simulink model "LogisticDelayed2"  (Simulink 6.6)
settings: Solver=ode45  StartTime=0.0  StopTime=60  RelTol=1e-3
settings Model: Creator=mxkana  LastModifiedBy=mxkana

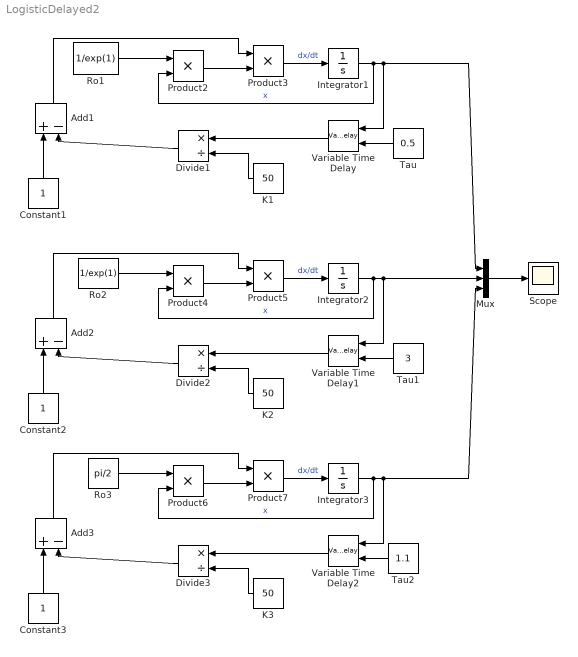
== system LogisticDelayed2 ==
  Add1 : Sum  Orientation=up  Inputs=+-  OutScaling=2^-10
  Add2 : Sum  Orientation=up  Inputs=+-  OutScaling=2^-10
  Add3 : Sum  Orientation=up  Inputs=+-  OutScaling=2^-10
  Constant1 : Constant  Orientation=up
  Constant2 : Constant  Orientation=up
  Constant3 : Constant  Orientation=up
  Divide1 : Product  Orientation=left  Inputs=*/  OutScaling=2^-10
  Divide2 : Product  Orientation=left  Inputs=*/  OutScaling=2^-10
  Divide3 : Product  Orientation=left  Inputs=*/  OutScaling=2^-10
  Integrator1 : Integrator  InitialCondition=1
  Integrator2 : Integrator  InitialCondition=1
  Integrator3 : Integrator  InitialCondition=1
  K1 : Constant  Orientation=left  Value=50
  K2 : Constant  Orientation=left  Value=50
  K3 : Constant  Orientation=left  Value=50
  Mux : Mux  Inputs=3
  Product{2..7} (6 alike) : Product  RndMeth=Zero
  Ro1 : Constant  Value=1/exp(1)
  Ro2 : Constant  Value=1/exp(1)
  Ro3 : Constant  Value=pi/2
  Scope : Scope
      settings: YMin=0  YMax=100
  Tau : Constant  Orientation=left  Value=0.5
  Tau1 : Constant  Orientation=left  Value=3
  Tau2 : Constant  Orientation=left  Value=1.1
  Variable Time Delay : VariableTransportDelay  Orientation=left  MaximumDelay=10
  Variable Time Delay1 : VariableTransportDelay  Orientation=left  MaximumDelay=10
  Variable Time Delay2 : VariableTransportDelay  Orientation=left  MaximumDelay=10
  wires:
  Constant1/1 -> Add1/1
  Ro1/1 -> Product2/1
  Product3/1 -> Integrator1/1  "dx/dt"
  Product2/1 -> Product3/2
  Integrator1/1 -> Product2/2, Variable Time Delay/1, Mux/1  "x"
  K1/1 -> Divide1/2
  Divide1/1 -> Add1/2
  Add1/1 -> Product3/1
  Tau/1 -> Variable Time Delay/2
  Variable Time Delay/1 -> Divide1/1
  Mux/1 -> Scope/1
  Constant2/1 -> Add2/1
  Ro2/1 -> Product4/1
  Product5/1 -> Integrator2/1  "dx/dt"
  Product4/1 -> Product5/2
  Integrator2/1 -> Product4/2, Variable Time Delay1/1, Mux/2  "x"
  K2/1 -> Divide2/2
  Divide2/1 -> Add2/2
  Add2/1 -> Product5/1
  Tau1/1 -> Variable Time Delay1/2
  Variable Time Delay1/1 -> Divide2/1
  Constant3/1 -> Add3/1
  Ro3/1 -> Product6/1
  Product7/1 -> Integrator3/1  "dx/dt"
  Product6/1 -> Product7/2
  Integrator3/1 -> Product6/2, Variable Time Delay2/1, Mux/3  "x"
  K3/1 -> Divide3/2
  Divide3/1 -> Add3/2
  Add3/1 -> Product7/1
  Tau2/1 -> Variable Time Delay2/2
  Variable Time Delay2/1 -> Divide3/1
